simulink model "dyn_dist_mpc_control_sim"  (R2019b)
settings: Solver=FixedStepAuto  StartTime=0.0  StopTime=71.45  FixedStep=h  RelTol=1e-3
values from neighbouring files (symbols this model uses):
  C_f = 710    [Copy_of_lateral_2_dof_model.m]    (also in init.m = 40000; init_scen_1.m = 40000; init_scen_3.m = 40000; lateral_2_dof_model.m = 1420)
  C_r = 710    [Copy_of_lateral_2_dof_model.m]    (also in init.m = 40000; init_scen_1.m = 40000; init_scen_3.m = 40000; lateral_2_dof_model.m = 1420)
  h = 0.1    [Example_9_Tracking_Delta_Input_Formulation.m]    (also in dyn_dist_mpc_control.m = 0.01; dyn_mpc_control.m = 0.01; dyn_pid_control.m = 0.01; init.m = 0.05)
  l_r = 100    [Copy_of_lateral_2_dof_model.m]    (also in init.m = 0.4125; init_scen_1.m = 0.4125; init_scen_3.m = 0.4125; lateral_2_dof_model.m = 0.4125)
  mass = evalin('base','mass')    [Nonlinear_model.m]    (also in init.m = 505; init_scen_1.m = 505; init_scen_3.m = 505; lateral_2_dof_model.m = 505)
  robot_vel = 3    [Example_9_Tracking_Delta_Input_Formulation.m]    (also in Nonlinear_model.m = evalin('base','robot_vel'); dyn_dist_mpc_control.m = 1; dyn_mpc_control.m = 1; dyn_pid_control.m = 1)
  wind_dist = [ 0 5 4]    [dyn_dist_mpc_control.m]
libraries: mpclib x1, autolibshared x1
settings Model: Creator=faaizz  LastModifiedBy=faaizz
settings SFSimCC: CustomCodeUndefinedFunction=UseInterfaceOnly

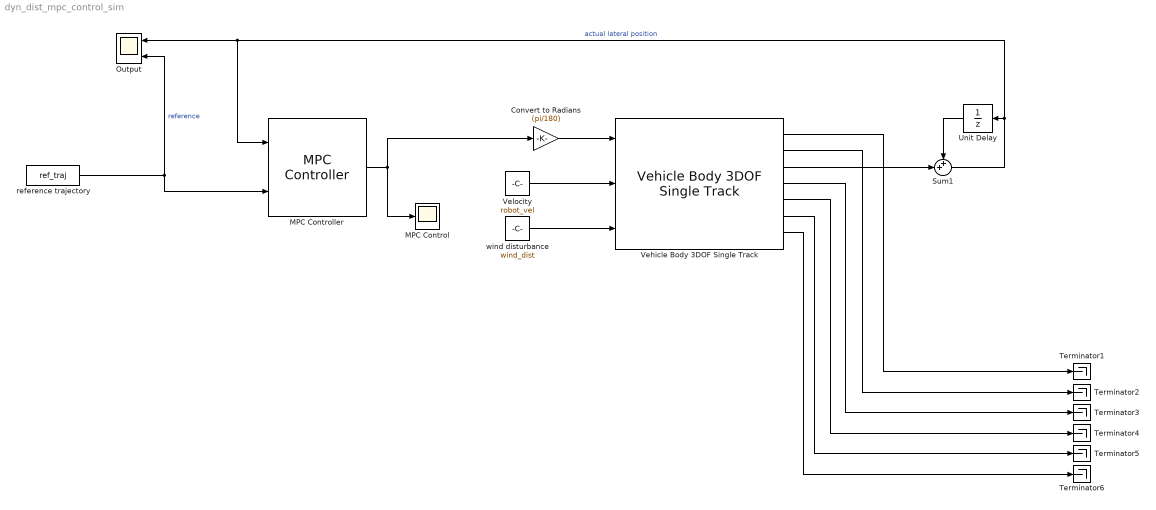
== system dyn_dist_mpc_control_sim ==
  Convert to Radians : Gain  Gain=(pi/180)
  MPC Control : Scope
  MPC Controller : mpclib/MPC Controller  SCDEnableBlockLinearizationSpecification=on  mpcobj=mpcobj  is_multiple=0  enable_value=0  return_u0=off  updateMPCinCallerWorkspace=on  md_inport=off  mv_inport=off  uref_inport=off  return_cost=off  return_mvseq=off  return_qpstatus=off  return_xseq=off  return_state=off  return_ovseq=off  state_inport=off  umin_inport=off  umax_inport=off  ymin_inport=off  ymax_inport=off  cc_inport=off  ywt_inport=off  uwt_inport=off  duwt_inport=off  rhoeps_inport=off  pm_inport=off  MaximumP=10  HorizonChoice=FixedHorizon  n_ts=0.01  n_p=50  n_mv=1  n_md=0  n_ud=0  n_mo=1  n_uo=0  BlockDataType=double  SampleTimeInherited=on  switch_inport=off
  Output : Scope  NumInputPorts=2
  Sum1 : Sum  Inputs=++|
  Terminator{1..6} (6 alike) : Terminator
  Unit Delay : UnitDelay  SampleTime=-1  HasFrameUpgradeWarning=on
  Vehicle Body 3DOF Single Track : autolibshared/Vehicle Body 3DOF Single Track  trackMode=Single (bicycle)  inputMode=External longitudinal velocity  frontSteerMode=on  rearSteerMode=off  windMode=on  muMode=off  extFMode=off  extMMode=off  extXo=off  extpsio=off  extxdoto=off  extro=off  extYo=off  extTamb=off  extydoto=off  aMode=2  NF=1  NR=2  m=mass  a=l_f  b=l_r  h=0.35/2  X_o=0  xdot_o=0  CalphaMode=off  sigmaMode=on  d=0  w=[1.4,1.4]  Cy_f=C_f*(180/pi)  Cy_r=C_r*(180/pi)  sigma_f=.1  sigma_r=.1  alpha_f_brk=[-.1 .1]  Cy_f_data=[-9e3 9e3]  alpha_r_brk=[-.1 .1]  Cy_r_data=[-9e3 9e3]  Y_o=0  ydot_o=0  Izz=I_zz  psi_o=0  r_o=0  Af=2  Cd=.3  Cl=.1  Cpm=.1  beta_w=[0:0.01:0.3]  Cs=[0:0.03:0.9]  Cym=[0:0.01:0.3]  Pabs=101325  Tair=273  g=9.81  mu=1  xdot_tol=.01  Fznom=5000  Fxtire_sat=7e4  Fytire_sat=7e4  longOff=0  latOff=0  vertOff=0  wrapAng=off
      settings: SourceProductName=Powertrain Blockset  SourceProductBaseCode=PW
  Velocity : Constant  Value=robot_vel
  reference trajectory : FromWorkspace  VariableName=ref_traj  SampleTime=h  OutputAfterFinalValue=Setting to zero
  wind disturbance : Constant  Value=wind_dist
  wires:
  reference trajectory/1 -> Output/2, MPC Controller/2  "reference"
  Velocity/1 -> Vehicle Body 3DOF Single Track/2
  MPC Controller/1 -> Convert to Radians/1, MPC Control/1
  Convert to Radians/1 -> Vehicle Body 3DOF Single Track/1
  Sum1/1 -> MPC Controller/1, Output/1, Unit Delay/1  "actual lateral position"
  Unit Delay/1 -> Sum1/1
  Vehicle Body 3DOF Single Track/3 -> Sum1/2
  wind disturbance/1 -> Vehicle Body 3DOF Single Track/3
  Vehicle Body 3DOF Single Track/1 -> Terminator1/1
  Vehicle Body 3DOF Single Track/2 -> Terminator2/1
  Vehicle Body 3DOF Single Track/4 -> Terminator3/1
  Vehicle Body 3DOF Single Track/5 -> Terminator4/1
  Vehicle Body 3DOF Single Track/6 -> Terminator5/1
  Vehicle Body 3DOF Single Track/7 -> Terminator6/1
